simulink model "SimulationMainModel"  (R2015b)
settings: Solver=ode15s  StartTime=0.0  StopTime=35  FixedStep=0.001  MinStep=1e-4  RelTol=1e-3
undefined symbols (not defined in the file or in its folder): bridge_final, camera, X, Y, Z
libraries: sm_lib x54, nesl_utility x18, simulatorLibrary x8, freescalecup_physmodlib x4, simulink x3, vrlib x1
(part 3 of 3)

== matlab function SimulationMainModel/Freescale Cup Car/Track/MATLAB Function ==
  data: s1 input; intersectionPoints output size=[4 2]; s2 input; track input; n output
function [ intersectionPoints, n ] = IntersectionPoint( s1, s2, track )
%UNTITLED Summary of this function goes here
%   Detailed explanation goes here
xs1 = s1(1);
ys1 = s1(2);

xs2 = s2(1);
ys2 = s2(2);

candidateIntersectionPoints = [NaN,NaN; NaN,NaN; NaN,NaN; NaN,NaN];

ipieceS1 = find(xs1>=track(:,1) & xs1<track(:,3) & ys1>=track(:,2) & ys1<track(:,4));
ipieceS2 = find(xs2>=track(:,1) & xs2<track(:,3) & ys2>=track(:,2) & ys2<track(:,4));

ipieceS1 = ipieceS1(1); % If I don't do this, Simulink will complain. Just replace
                        % the one-element ipieceS1 vector with its only
                        % element
ipieceS2 = ipieceS2(1);

n = 0;  % Number of intersections found

trackPieceS1 = track(ipieceS1,5);
trackPieceS2 = track(ipieceS2,5);
% In this if block, we compute the intersections between the infinite line
% that contains the camera view and the curve contained into the bounding
% box where S1 is.
% In this if block, check if the computed intersections are inside the
% bounding box where S1 is
if trackPieceS1==1 % vertical straight piece
    % Compute the coordinates of the intersection
    % The x coordinate of the straight line is in column 6
    candidateIntersectionPoints(n+1,1) = track(ipieceS1,6);
    
    % Equation of the line containing the camera view:
    % y = ys1 + (ys2-ys1)/(xs2-xs1)*(x-xs1)
    candidateIntersectionPoints(n+1,2) = ys1 + (ys2-ys1)/(xs2-xs1)*(candidateIntersectionPoints(1,1)-xs1);
    
    % Check if the intersection point is inside the bounding box. If so,
    % increase the number of intersections
    if(candidateIntersectionPoints(n+1,1)>=track(ipieceS1,1) && candidateIntersectionPoints(n+1,1)<track(ipieceS1,3) &&...
        candidateIntersectionPoints(n+1,2)>=track(ipieceS1,2) && candidateIntersectionPoints(n+1,2)<track(ipieceS1,4))
        n = n+1;
    end
    
elseif trackPieceS1==0 % horizontal straight piece
    % The y coordinate of the straight line is in column 6
    candidateIntersectionPoints(1,2) = track(ipieceS1,6);

    % Equation of the line containing the camera view:
    % x = xs1 + (xs2-xs1)/(ys2-ys1)*(y-ys1)
    candidateIntersectionPoints(1,1) = xs1 + (xs2-xs1)/(ys2-ys1)*(candidateIntersectionPoints(1,2)-ys1);

    if(candidateIntersectionPoints(n+1,1)>=track(ipieceS1,1) && candidateIntersectionPoints(n+1,1)<track(ipieceS1,3) &&...
        candidateIntersectionPoints(n+1,2)>=track(ipieceS1,2) && candidateIntersectionPoints(n+1,2)<track(ipieceS1,4))
        n = n+1;
    end
    
elseif trackPieceS1==2 % turn
    % Using the formulae at http://math.stackexchange.com/questions/228841/how-do-i-calculate-the-intersections-of-a-straight-line-and-a-circle
    if(xs2-xs1>eps) % Condition equivalent to xs2~=xs1 for finite precision
        m = (ys2-ys1)/(xs2-xs1);
        c = ys1 - xs1*m;
        r = track(ipieceS1,6); % for turns, radius is in column 6
        p = track(ipieceS1,7); % center coordinates are in columns 7 and 8
        q = track(ipieceS1,8);
        
        A = m*m+1;
        B = 2*(m*c-m*q-p);
        C = q*q - r*r + p*p -2*c*q + c*c;
        delta = B*B-4*A*C;
        % There are two intersection points (possibly coincident) only when delta>=0
        if(delta>=0)
            candidateIntersectionPoints(n+1,1) = (-B+sqrt(delta))/(2*A);
            candidateIntersectionPoints(n+1,2) = m*candidateIntersectionPoints(n+1,1)+c;
            if(candidateIntersectionPoints(n+1,1)>=track(ipieceS1,1) && candidateIntersectionPoints(n+1,1)<track(ipieceS1,3) &&...
                candidateIntersectionPoints(n+1,2)>=track(ipieceS1,2) && candidateIntersectionPoints(n+1,2)<track(ipieceS1,4))
                n = n+1;
            end
            % Second intersection
            candidateIntersectionPoints(n+1,1) = (-B-sqrt(delta))/(2*A);
            candidateIntersectionPoints(n+1,2) = m*candidateIntersectionPoints(n+1,1)+c;
            if(candidateIntersectionPoints(n+1,1)>=track(ipieceS1,1) && candidateIntersectionPoints(n+1,1)<track(ipieceS1,3) &&...
                candidateIntersectionPoints(n+1,2)>=track(ipieceS1,2) && candidateIntersectionPoints(n+1,2)<track(ipieceS1,4))
                n = n+1;
            end
        end
    else %The camera view segment is (approximately) vertical
        r = track(ipieceS1,6);
        A = 1;
        B = -2*track(ipieceS1,8);
        C = (xs1-track(ipieceS1,7))*(xs1-track(ipieceS1,7))-r*r;
        delta = B*B-4*A*C;
        if(delta>=0)
            candidateIntersectionPoints(n+1,1)=xs1;
            candidateIntersectionPoints(n+1,2)= (-B+sqrt(delta))/(2*A);
            if(candidateIntersectionPoints(n+1,1)>=track(ipieceS1,1) && candidateIntersectionPoints(n+1,1)<track(ipieceS1,3) &&...
                candidateIntersectionPoints(n+1,2)>=track(ipieceS1,2) && candidateIntersectionPoints(n+1,2)<track(ipieceS1,4))
                n = n+1;
            end
            
            candidateIntersectionPoints(n+1,1)=xs1;
            candidateIntersectionPoints(n+1,2)= (-B-sqrt(delta))/(2*A);
            if(candidateIntersectionPoints(n+1,1)>=track(ipieceS1,1) && candidateIntersectionPoints(n+1,1)<track(ipieceS1,3) &&...
                candidateIntersectionPoints(n+1,2)>=track(ipieceS1,2) && candidateIntersectionPoints(n+1,2)<track(ipieceS1,4))
                n = n+1;
            end
        end
    end
end


% If the two endpoints of the camera view are in different bounding boxes,
% check the second bounding box
if(ipieceS2~=ipieceS1)
    if trackPieceS2==1 % vertical straight piece
        % Compute the coordinates of the intersection
        % The x coordinate of the straight line is in column 6
        candidateIntersectionPoints(n+1,1) = track(ipieceS2,6);

        % Equation of the line containing the camera view:
        % y = ys1 + (ys2-ys1)/(xs2-xs1)*(x-xs1)
        candidateIntersectionPoints(n+1,2) = ys1 + (ys2-ys1)/(xs2-xs1)*(candidateIntersectionPoints(1,1)-xs1);

        % Check if the intersection point is inside the bounding box. If so,
        % increase the number of intersections
        if(candidateIntersectionPoints(n+1,1)>=track(ipieceS2,1) && candidateIntersectionPoints(n+1,1)<track(ipieceS2,3) &&...
            candidateIntersectionPoints(n+1,2)>=track(ipieceS2,2) && candidateIntersectionPoints(n+1,2)<track(ipieceS2,4))
            n = n+1;
        end

    elseif trackPieceS2==0 % horizontal straight piece
        % The y coordinate of the straight line is in column 6
        candidateIntersectionPoints(1,2) = track(ipieceS1,6);

        % Equation of the line containing the camera view:
        % x = xs1 + (xs2-xs1)/(ys2-ys1)*(y-ys1)
        candidateIntersectionPoints(1,1) = xs1 + (xs2-xs1)/(ys2-ys1)*(candidateIntersectionPoints(1,2)-ys1);

        if(candidateIntersectionPoints(n+1,1)>=track(ipieceS2,1) && candidateIntersectionPoints(n+1,1)<track(ipieceS2,3) &&...
            candidateIntersectionPoints(n+1,2)>=track(ipieceS2,2) && candidateIntersectionPoints(n+1,2)<track(ipieceS2,4))
            n = n+1;
        end

    elseif trackPieceS2==2 % turn
        % Using the formulae at http://math.stackexchange.com/questions/228841/how-do-i-calculate-the-intersections-of-a-straight-line-and-a-circle
        if(xs2-xs1>eps) % Condition equivalent to xs2~=xs1 for finite precision
            m = (ys2-ys1)/(xs2-xs1);
            c = ys1 - xs1*m;
            r = track(ipieceS2,6); % for turns, radius is in column 6
            p = track(ipieceS2,7); % center coordinates are in columns 7 and 8
            q = track(ipieceS2,8);

            A = m*m+1;
            B = 2*(m*c-m*q-p);
            C = q*q - r*r + p*p -2*c*q + c*c;
            delta = B*B-4*A*C;
            % There are two intersection points (possibly coincident) only when delta>=0
            if(delta>=0)
                candidateIntersectionPoints(n+1,1) = (-B+sqrt(delta))/(2*A);
                candidateIntersectionPoints(n+1,2) = m*candidateIntersectionPoints(n+1,1)+c;
                if(candidateIntersectionPoints(n+1,1)>=track(ipieceS2,1) && candidateIntersectionPoints(n+1,1)<track(ipieceS2,3) &&...
                    candidateIntersectionPoints(n+1,2)>=track(ipieceS2,2) && candidateIntersectionPoints(n+1,2)<track(ipieceS2,4))
                    n = n+1;
                end
                % Second intersection
                candidateIntersectionPoints(n+1,1) = (-B-sqrt(delta))/(2*A);
                candidateIntersectionPoints(n+1,2) = m*candidateIntersectionPoints(n+1,1)+c;
                if(candidateIntersectionPoints(n+1,1)>=track(ipieceS2,1) && candidateIntersectionPoints(n+1,1)<track(ipieceS2,3) &&...
                    candidateIntersectionPoints(n+1,2)>=track(ipieceS2,2) && candidateIntersectionPoints(n+1,2)<track(ipieceS2,4))
                    n = n+1;
                end
            end
        else %The camera view segment is (approximately) vertical
            r = track(ipieceS1,6);
            A = 1;
            B = -2*track(ipieceS1,8);
            C = (xs1-track(ipieceS1,7))*(xs1-track(ipieceS1,7))-r*r;
            delta = B*B-4*A*C;
            if(delta>=0)
                candidateIntersectionPoints(n+1,1)=xs1;
                candidateIntersectionPoints(n+1,2)= (-B+sqrt(delta))/(2*A);
                if(candidateIntersectionPoints(n+1,1)>=track(ipieceS2,1) && candidateIntersectionPoints(n+1,1)<track(ipieceS2,3) &&...
                    candidateIntersectionPoints(n+1,2)>=track(ipieceS2,2) && candidateIntersectionPoints(n+1,2)<track(ipieceS2,4))
                    n = n+1;
                end

                candidateIntersectionPoints(n+1,1)=xs1;
                candidateIntersectionPoints(n+1,2)= (-B-sqrt(delta))/(2*A);
                if(candidateIntersectionPoints(n+1,1)>=track(ipieceS2,1) && candidateIntersectionPoints(n+1,1)<track(ipieceS2,3) &&...
                    candidateIntersectionPoints(n+1,2)>=track(ipieceS2,2) && candidateIntersectionPoints(n+1,2)<track(ipieceS2,4))
                    n = n+1;
                end
            end
        end
    end
end

% Last check. Check if the points found so far are in the camera view
% segment. Exclude the others
% The following line must be read as follows. Take only the intersection
% points (= the rows in candidateIntersectionPoints) whose x coordinate (= the element
% in column 1 of each row) lies between the x coordinate of S1 and the x
% coordinate of S2. Overwrite the old points in candidateIntersectionPoints.
intersectionPoints = [NaN NaN; NaN NaN; NaN NaN; NaN NaN];
candidateIntersectionPoints = candidateIntersectionPoints(candidateIntersectionPoints(:,1)>=xs1 & candidateIntersectionPoints(:,1)<=xs2,:);
[n,~] = size(candidateIntersectionPoints);
intersectionPoints(1:n,:) = candidateIntersectionPoints;


end

== matlab function SimulationMainModel/Freescale Cup Car/Camera Subsystem/MATLAB Function1 ==
  data: u input; y output
function y = axesSimscape2VR(u)
%#codegen

y = zeros(3,1);
y(1) = -u(1);
y(2) = u(3);
y(3) = u(2);

== matlab function SimulationMainModel/Simple Image Processing/MATLAB Function ==
  data: u input; y output
function y = fromIndexToPosition(u)
%#codegen

y = - u + 64;

== matlab function SimulationMainModel/Simple Image Processing/Signal_Proc ==
  data: centerIdx output; camData input
function centerIdx  = centerTrackIdx(camData)

threshold = (max(camData)+min(camData))/2;
black = find(camData<threshold);
if(length(black)>=2)
    centerIdx = black(floor(length(black)/2));
else
    centerIdx = 64;
end

%%%%%%%%%%%%%%%%%%%%%%%%%%%%%%%%%%%%%%%%%%%%%%%%%%%%%%%%%%%%%%%%%%%%%%%%%%%%%%%%%%%

%find STOP
% 
% h = 29;%camera high
% a = 29.21;%cm (3'-1/2") length from lateral line to center track
% b=60;
% camera_error = 7;
% d = sqrt(b^2+h^2);%diagonal length from camera to view center point
% alfa = atan2(a,d);%optical angle from center to lateral line
% pixel_gap = round(alfa/0.007604262);%pixel from lateral line to center track
% pixel_edge = 64 - pixel_gap + camera_error;%pixel from lateral line to outdoor track
% s1 = 3.81;%cm [1 1/2"] center track to begin stop
% s2 = 13.97;%cm [5 1/2"] center track to end stop
% alfa1 = atan2(s1,d);
% alfa2 = atan2(s2,d);
% s1_pixel = round(alfa1/0.007604262);
% s2_pixel = round(alfa2/0.007604262);
% 
% 
% 
% %         if length(find(camData(64-s2_pixel:64-s1_pixel) < threshold)) > 0.1*(s2_pixel-s1_pixel) &&...
% %             length(find(camData(64+s1_pixel:64+s2_pixel) < threshold)) > 0.1*(s2_pixel-s1_pixel) &&...
% %             length(find(camData(64-s1_pixel:64+s1_pixel) > threshold)) > 0.1*2*s1_pixel
% 
% if length(find(camData(64-s2_pixel-10:64-s1_pixel+10) < threshold)) > 0.6*(s2_pixel-s1_pixel) &&...
%     length(find(camData(64+s1_pixel-10:64+s2_pixel+10) < threshold)) > 0.6*(s2_pixel-s1_pixel) &&...
%     length(find(camData(64-s1_pixel-10:64+s1_pixel+10) > threshold)) > 2*s1_pixel
% 
% %         if length(find(camData(30:98) < threshold)) > (s2_pixel-s1_pixel) &&...
% %             length(find(camData(64-s1_pixel:64+s1_pixel) > threshold)) > 0.1*2*s1_pixel
% 
%     stop = 1;
%     centerIdx=64;
% end
% 
% if length(find(camData(40:60) < threshold)) > 0.55*20 &&...
%     length(find(camData(70:90) < threshold)) > 0.55*20 &&...
%     length(find(camData(60:70) > threshold)) > 0.55*10
% 
% %         if length(find(camData(30:98) < threshold)) > (s2_pixel-s1_pixel) &&...
% %             length(find(camData(64-s1_pixel:64+s1_pixel) > threshold)) > 0.1*2*s1_pixel
% 
%     stop = 1;
%     centerIdx=64;
% end
